simulink model "Modelo_LeyDeControlMinima"  (R2026a)
settings: Solver=VariableStepAuto
values from neighbouring files (symbols this model uses):
  L_q = 5.8e-3    (= 0.0058)    [coeficientes.m]
  Pp = 3    [coeficientes.m]
libraries: eeTransforms x1
settings Model: Creator=barrios14101  LastModifiedBy=admin

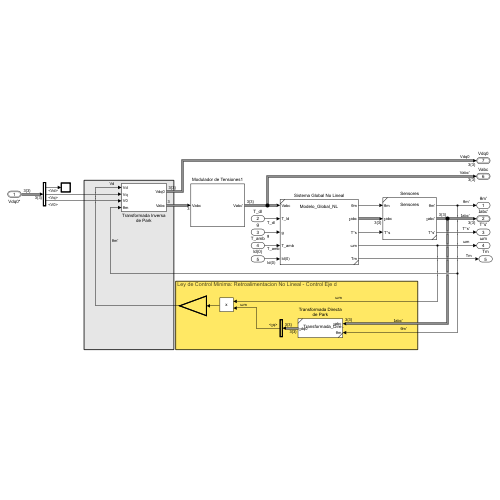
[thumbnail: Simulink's stored preview of the top-level diagram]
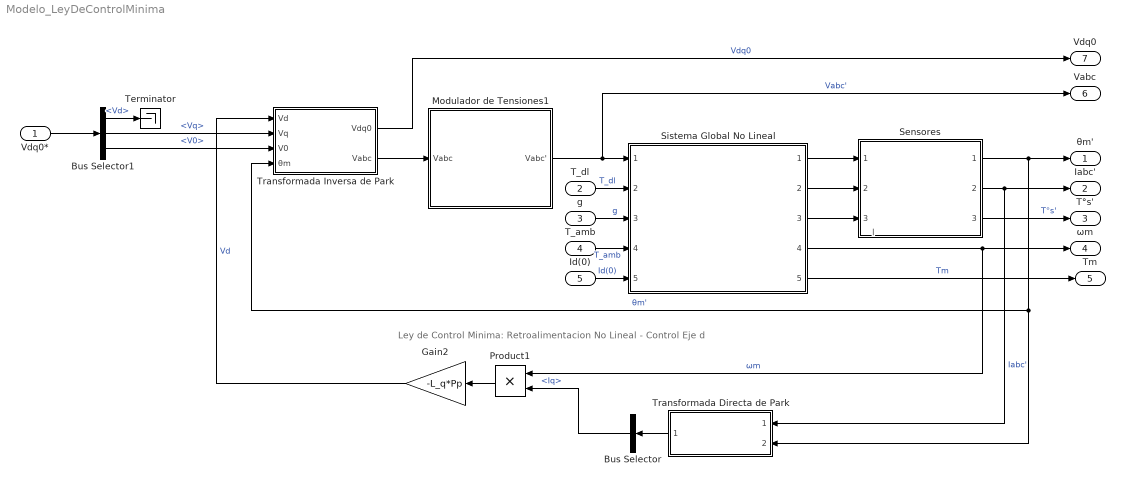
== system Modelo_LeyDeControlMinima ==
  note: Ley de Control Minima: Retroalimentacion No Lineal - Control Eje d
  note: Ⅰ
  Vdq0* : Inport  OutDataTypeStr=Bus: Vdq0
  T_dl : Inport  Port=2
  g : Inport  Port=3
  T_amb : Inport  Port=4
  Id(0) : Inport  Port=5
  Bus Selector : BusSelector  OutputSignals=Ⅰq
  Bus Selector1 : BusSelector  OutputSignals=Vd,Vq,V0
  Gain2 : Gain  Gain=-L_q*Pp
  Modulador de Tensiones1 : Subsystem
  Product1 : Product
  Sensores : Subsystem  ReferencedSubsystem=Sensores
  Sistema Global No Lineal : Subsystem  ReferencedSubsystem=Modelo_Global_NL
  Terminator : Terminator
  Transformada Directa de Park : Subsystem  ReferencedSubsystem=Transformada_Directa_de_Park_I
  Transformada Inversa de Park : Subsystem
  θm' : Outport
  Ⅰabc' : Outport  Port=2  OutDataTypeStr=Bus: Iabc
  T°s' : Outport  Port=3
  ωm : Outport  Port=4
  Tm : Outport  Port=5
  Vabc : Outport  Port=6  OutDataTypeStr=Bus: Vabc
  Vdq0 : Outport  Port=7  OutDataTypeStr=Bus: Vdq0
  wires:
  Sensores/1 -> Transformada Inversa de Park/4(θm), Transformada Directa de Park/2, θm'/1  "θm'"
  Sistema Global No Lineal/4 -> Product1/1, ωm/1  "ωm"
  Gain2/1 -> Transformada Inversa de Park/1(Vd)  "Vd"
  Sensores/2 -> Transformada Directa de Park/1, Ⅰabc'/1  "Ⅰabc'"
  Product1/1 -> Gain2/1
  Transformada Inversa de Park/2(Vabc) -> Modulador de Tensiones1/1(Vabc)
  Bus Selector/1 -> Product1/2  "<Ⅰq>"
  Transformada Directa de Park/1 -> Bus Selector/1
  Modulador de Tensiones1/1(Vabc') -> Sistema Global No Lineal/1, Vabc/1  "Vabc'"
  Sistema Global No Lineal/2 -> Sensores/2
  Sistema Global No Lineal/3 -> Sensores/3
  Sistema Global No Lineal/1 -> Sensores/1
  Sistema Global No Lineal/5 -> Tm/1  "Tm"
  Sensores/3 -> T°s'/1  "T°s'"
  Transformada Inversa de Park/1(Vdq0) -> Vdq0/1  "Vdq0"
  Vdq0*/1 -> Bus Selector1/1
  T_dl/1 -> Sistema Global No Lineal/2  "T_dl"
  T_amb/1 -> Sistema Global No Lineal/4  "T_amb"
  g/1 -> Sistema Global No Lineal/3  "g"
  Bus Selector1/1 -> Terminator/1  "<Vd>"
  Bus Selector1/2 -> Transformada Inversa de Park/2(Vq)  "<Vq>"
  Bus Selector1/3 -> Transformada Inversa de Park/3(V0)  "<V0>"
  Id(0)/1 -> Sistema Global No Lineal/5  "Id(0)"

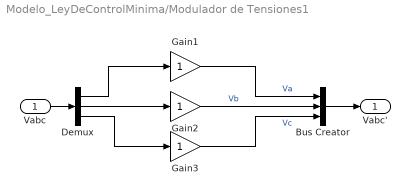
== system Modelo_LeyDeControlMinima/Modulador de Tensiones1 ==
  Vabc : Inport
  Bus Creator : BusCreator  Inputs=3
  Demux : Demux  Outputs=3
  Gain1 : Gain
  Gain2 : Gain
  Gain3 : Gain
  Vabc' : Outport
  wires:
  Gain2/1 -> Bus Creator/2  "Vb"
  Gain3/1 -> Bus Creator/3  "Vc"
  Gain1/1 -> Bus Creator/1  "Va"
  Demux/2 -> Gain2/1
  Vabc/1 -> Demux/1
  Demux/1 -> Gain1/1
  Demux/3 -> Gain3/1
  Bus Creator/1 -> Vabc'/1

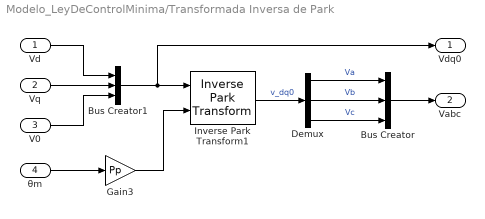
== system Modelo_LeyDeControlMinima/Transformada Inversa de Park ==
  Vd : Inport
  Vq : Inport  Port=2
  V0 : Inport  Port=3
  θm : Inport  Port=4
  Bus Creator : BusCreator  Inputs=3
  Bus Creator1 : BusCreator  Inputs=3
  Demux : Demux  Outputs=3
  Gain3 : Gain  Gain=Pp
  Inverse Park Transform1 : eeTransforms/Inverse Park Transform  AxisAlignment=Q-axis  PowerInvariant=off
      settings: LibrarySourceBlock=|
      | ee_sl_lib/Mathematical
      | Transforms/Inverse
      | Park Transform
  Vdq0 : Outport
  Vabc : Outport  Port=2
  wires:
  Gain3/1 -> Inverse Park Transform1/2
  Inverse Park Transform1/1 -> Demux/1  "v_dq0"
  Demux/1 -> Bus Creator/1  "Va"
  Demux/3 -> Bus Creator/3  "Vc"
  Demux/2 -> Bus Creator/2  "Vb"
  Bus Creator/1 -> Vabc/1
  θm/1 -> Gain3/1
  Vd/1 -> Bus Creator1/1
  Vq/1 -> Bus Creator1/2
  V0/1 -> Bus Creator1/3
  Bus Creator1/1 -> Inverse Park Transform1/1, Vdq0/1
